simulink model "cable_model"  (R2020a)
settings: Solver=ode4  StartTime=0.0  StopTime=100  FixedStep=0.0001  RelTol=1e-3
values from neighbouring files (symbols this model uses):
  d = 0.01    [cable_model_matlab.m]    (also in parameters.m; umbilical_model.m; umbilical_model_simulink.m)
  g = [0,0,9.81]    [cable_model_matlab.m]    (also in parameters.m; umbilical_model.m; umbilical_model_simulink.m)
  k = n+1    [cable_model_matlab.m]    (also in parameters.m = int32(n+1); umbilical_model.m = 6; umbilical_model_simulink.m = 21)
  l0 = lc/n    [cable_model_matlab.m]    (also in parameters.m = 1; umbilical_model.m = 4; umbilical_model_simulink.m)
  m = eye(3)*mc/n    [cable_model_matlab.m]    (also in parameters.m; umbilical_model.m; umbilical_model_simulink.m)
  rho = 1020    [cable_model_matlab.m]    (also in parameters.m; umbilical_model.m; umbilical_model_simulink.m)
settings Model: Creator=mikafabricius  LastModifiedBy=mikafabricius

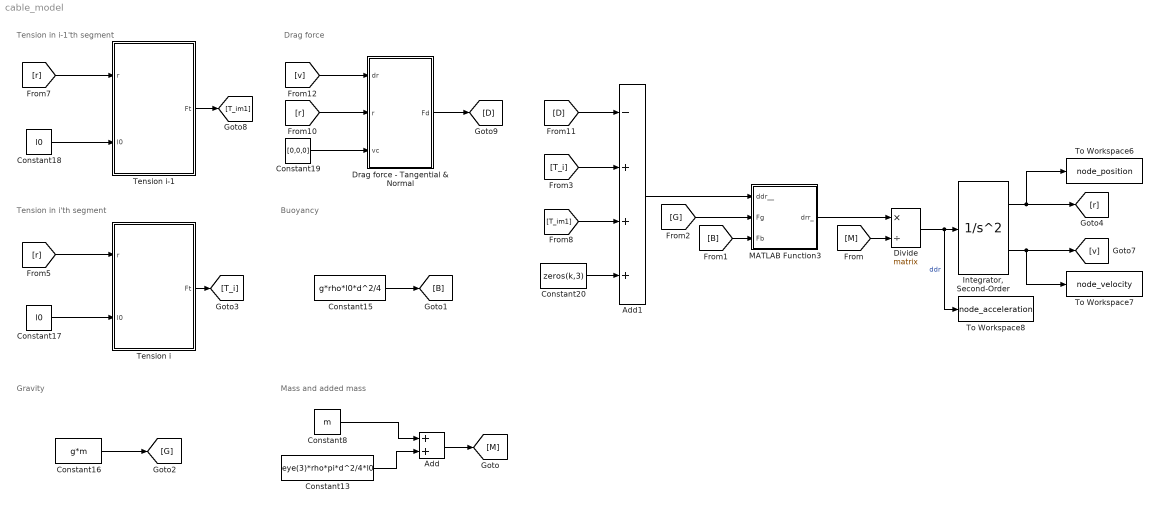
== system cable_model ==
  note: Gravity
  note: Tension in i-1'th segment
  note: Mass and added mass
  note: Tension in i'th segment
  note: Buoyancy
  note: Drag force
  Add : Sum
  Add1 : Sum  Inputs=-+++
  Constant13 : Constant  Value=eye(3)*rho*pi*d^2/4*l0
  Constant15 : Constant  Value=g*rho*l0*d^2/4  VectorParams1D=off
  Constant16 : Constant  Value=g*m  VectorParams1D=off
  Constant17 : Constant  Value=l0
  Constant18 : Constant  Value=l0
  Constant19 : Constant  Value=[0,0,0]  VectorParams1D=off
  Constant20 : Constant  Value=zeros(k,3)
  Constant8 : Constant  Value=m
  Divide : Product  Inputs=*/  Multiplication=Matrix(*)
  Drag force - Tangential & Normal : MATLAB Function  TreatAsAtomicUnit=on
  "Integrator, Second-Order" : SecondOrderIntegrator  ICX=r_ini_i  ICDXDT=v_ini_i
  MATLAB Function3 : MATLAB Function  TreatAsAtomicUnit=on
  Tension i : MATLAB Function  TreatAsAtomicUnit=on
  Tension i-1 : MATLAB Function  TreatAsAtomicUnit=on
  To Workspace6 : ToWorkspace  VariableName=node_position  SaveFormat=Structure With Time  SampleTime=-1
  To Workspace7 : ToWorkspace  VariableName=node_velocity  SaveFormat=Structure With Time  SampleTime=-1
  To Workspace8 : ToWorkspace  VariableName=node_acceleration  SaveFormat=Structure With Time  SampleTime=-1
  wires:
  Drag force - Tangential & Normal/1(Fd) -> [D]
  [r] -> Tension i/1(r)
  Add/1 -> [M]
  [M] -> Divide/2
  [T_i] -> Add1/2
  Constant18/1 -> Tension i-1/2(l0)
  Divide/1 -> To Workspace8/1, "Integrator, Second-Order"/1  "ddr"
  Constant15/1 -> [B]
  [D] -> Add1/1
  "Integrator, Second-Order"/2 -> [v], To Workspace7/1
  [T_im1] -> Add1/3
  [r] -> Tension i-1/1(r)
  [r] -> Drag force - Tangential & Normal/2(r)
  MATLAB Function3/1(drr_) -> Divide/1
  Constant19/1 -> Drag force - Tangential & Normal/3(vc)
  [v] -> Drag force - Tangential & Normal/1(dr)
  Constant17/1 -> Tension i/2(l0)
  Constant8/1 -> Add/1
  Tension i-1/1(Ft) -> [T_im1]
  Constant16/1 -> [G]
  Tension i/1(Ft) -> [T_i]
  Add1/1 -> MATLAB Function3/1(ddr__)
  "Integrator, Second-Order"/1 -> To Workspace6/1, [r]
  [B] -> MATLAB Function3/3(Fb)
  Constant13/1 -> Add/2
  Constant20/1 -> Add1/4
  [G] -> MATLAB Function3/2(Fg)

== matlab function cable_model/MATLAB Function3 ==
  data: ddr__ input; drr_ output; Fg input; Fb input
function drr_ = fcn(ddr__,Fg,Fb)
drr_ = zeros(length(ddr__),3);
for i=1:length(ddr__)
    drr_(i,:) = ddr__(i,:) + Fb - Fg;
    if i == 1
        drr_(i,:) = [0,0,0];
    end
end

== matlab function cable_model/Tension i ==
  data: r input; Ft output; l0 input
function Ft = tension(r,l0)
Ft = zeros(length(r),3);
    for i=1:length(r)
        E = 200*10^9; % Pa, kg/(m*s^2), Young's modulus
        d = 0.01; % m, diameter of umbilical
        if i == 1 || i == 21
            Ft(i,:) = [0,0,0];
        else
            Ft(i,:) = pi*d^2/4*E*(norm(r(i+1,:)-r(i,:))-l0)/l0*(r(i+1,:)-r(i,:))/(norm(r(i+1,:)-r(i,:)));
        end
    end
end

== matlab function cable_model/Tension i-1 ==
  data: r input; Ft output; l0 input
function Ft = tension(r,l0)
    Ft = zeros(length(r),3);
    for i=1:length(r)
        E = 200*10^9; % Pa, kg/(m*s^2), Young's modulus
        d = 0.01; % m, diameter of umbilical
        if i == 1
            Ft(i,:) = [0,0,0];
        else
            Ft(i,:) = pi*d^2/4*E*(norm(r(i-1,:)-r(i,:))-l0)/l0*(r(i-1,:)-r(i,:))/(norm(r(i-1,:)-r(i,:)));
        end
    end
end

== matlab function cable_model/Drag force - Tangential & Normal ==
  data: dr input; r input; Fd output; vc input
function Fd = drag(dr,r,vc)
   Fd = zeros(length(r),3);
   for i=1:length(r)
        
        rho = 1020; % kg/m^3, density of seawater
        d = 0.01; % m, diameter of umbilical
        Ct = 0.2; % Tangential drag coefficient
        Cn = 0.2; % Normal drag coefficient
        
        if i == 1
            Fd(i,:) = [0,0,0];
        else
            if i == 21
                t = (r(i,:)-r(i-1,:))/norm(r(i,:)-r(i-1,:));
            else
                t = (r(i+1,:)-r(i,:))/norm(r(i+1,:)-r(i,:));
            end
            D_t = 1/2*rho*Ct*norm(r(i-1,:)+r(i,:))*d*((dr(i,:)-vc).*t).^2;
            D_n = pi/8*rho*d^2*Cn*((dr(i,:)-vc)-(dr(i,:)-vc).*t).^2;
            Fd(i,:) = D_t + D_n;
            Fd(i,:) = Fd(i,:) .* sign(dr(i,:));
        end
    end
end
